simulink model "estimation_mdl"  (R2022b)
settings: Solver=FixedStepDiscrete  StartTime=0.0  StopTime=100  FixedStep=.1  RelTol=1e-3
values from neighbouring files (symbols this model uses):
  H = [1 3;4 0]    [estimation2d.m]    (also in estimation3d.m = [1 0 0;0 1 0;2 0 3]; filtering2_s.m = [1 3 -2;4 4 0]; tst1.m = [1 1])
  m = size(H,1)    [estimation2d.m]    (also in estimation3d.m; tst1.m)
  P0 = 1e2*eye(2)    [estimation2d.m]    (also in estimation3d.m = 1e2*eye(3); filtering1_s.m = V*diag([1 2])/V; filtering2_s.m = 1e1*eye(3); tst1.m = V*sqrt(D)*V.')
  Q = V*sqrt(D)    [estimation2d.m]    (also in estimation3d.m; ex_3_11.m = V*D12; filtering1_s.m; filtering2_s.m)
  R = (V /(sqrt(L))).'    [cellipse.m]    (also in estimation2d.m = V*D/V; estimation3d.m = V*D/V; filtering1_s.m = 3; filtering2_s.m = V*D/V)
  Ri = V*sqrt(L)    [cellipse.m]    (also in estimation2d.m = inv(R); estimation3d.m = inv(R); filtering1_s.m = inv(R); filtering2_s.m = inv(R))
  theta = 0:.05:2*pi    [cellipse.m]    (also in estimation2d.m = [8;-3]; estimation3d.m = [8;-3;4]; filtering1_s.m = [1.2, 3.4]; filtering2_s.m = [8;-3;15])
  xhat0 = [-5;-5]    [estimation2d.m]    (also in estimation3d.m = [-5;-5;0]; filtering1_s.m = [1;1]; filtering2_s.m = [0;0;0]; tst1.m)
undefined symbols (not defined in the file or in its folder): Discrete, Time
libraries: dspinverses x2, ctrlSharedLib x2
settings Model: Creator=hp_desktop  LastModifiedBy=hp_desktop

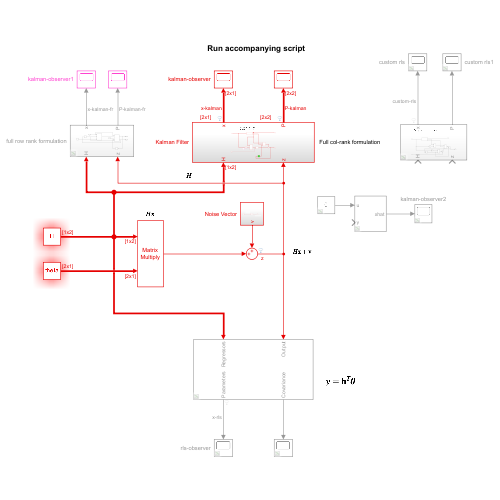
[thumbnail: Simulink's stored preview of the top-level diagram]
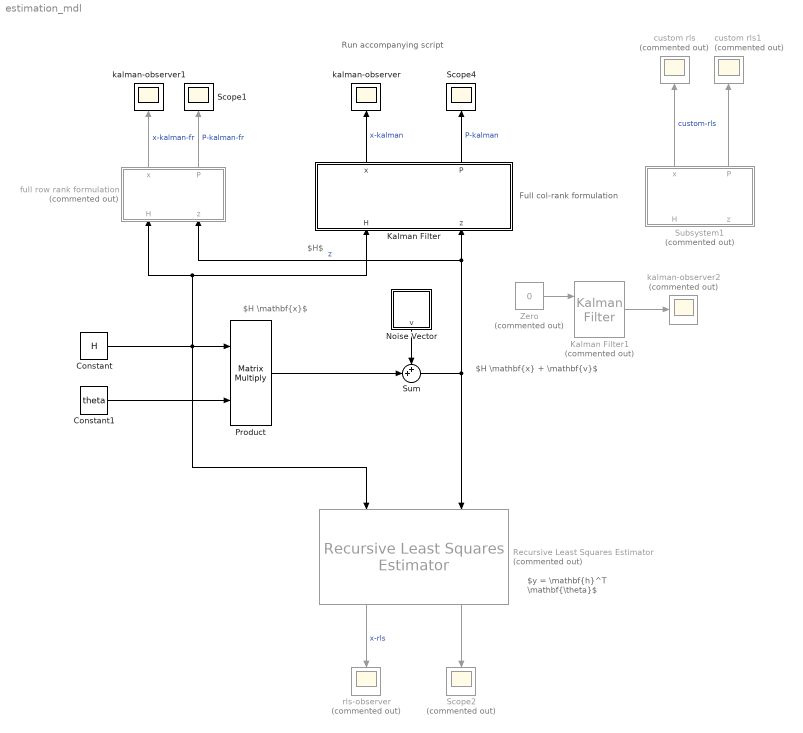
== system estimation_mdl ==
  note: Full col-rank formulation
  note: $H \mathbf{x}$
  note: Run accompanying script
  note: $y = \mathbf{h}^T \mathbf{\theta}$
  note: $H$
  note: $H \mathbf{x} + \mathbf{v}$
  Constant : Constant  Value=H  VectorParams1D=off  SampleTime=-1
  Constant1 : Constant  Value=theta  VectorParams1D=off  SampleTime=-1
  Kalman Filter : Subsystem
  Kalman Filter1 : ctrlSharedLib/Kalman Filter  Commented=on  TimeDomain=Discrete-Time  UseCurrentEstimator=on  ModelSource=Individual A, B, C, D matrices  ModelSourceVariable=ss(0.95,1,1,0,1)  A=[0 0;0 0]  B=[0;0]  C=H  D=zeros(m,1)  NumberOfStates=1  NumberOfInputs=1  NumberOfOutputs=1  InitialEstimateSource=Dialog  X0=xhat0  P0=10  UseK=off  UseGH=off  NumberOfProcessNoiseInputs=1  G=1  TimeInvariantG=on  H=0  TimeInvariantH=on  Q=0  TimeInvariantQ=on  R=R  TimeInvariantR=on  N=0  TimeInvariantN=on  AddInputPort=on  AddEnablePort=off  OutputEstimatedY=off  OutputP=off  Ts=-1
  Noise Vector : Subsystem
  Product : Product  Multiplication=Matrix(*)
  Recursive Least Squares Estimator : ctrlSharedLib/Recursive Least Squares Estimator  Commented=on  InitialEstimateSource=Internal  InitialParameterData=xhat0  P0=P0  InitialRegressors=0  InitialOutputs=0  History=Infinite  WindowLength=200  EstimationMethod=Kalman Filter  AdaptationParameter=0  HasTimeVaryingAdaptationParameter=off  NormalizationBias=eps  OutputError=off  OutputP=on  AddEnablePort=off  InputProcessing=Frame-based  Ts=-1
      settings: LibrarySourceBlock=slident/Estimators/Recursive Least Squares Estimator
  Scope1 : Scope
  Scope2 : Scope  Commented=on
  Scope4 : Scope
  Subsystem1 : Subsystem  Commented=on
      settings: PortSchema="{\"entries\":[{\"content\":{\"sides\":[{\"content\":{\"connectorIds\":[]},\"type\":\"ConnectorPlacement.EquallySpacedRectSide\",\"uuid\":\"bee4a480-fac8-4835-b5c1-70eb87c43e95\"},{\"content\":{\"connectorIds\":[],\"side\":\"RIGHT\"},\"type\":\"ConnectorPlacement.EquallySpacedRectSide\",\"uuid\":\"cb84ae2e-f606-4d86-aba4-d3e87a068395\"},{\"content\":{\"connectorIds\":[\"Out1\",\"Out2\"],\"side\":\"TOP\"},\"type\":\"ConnectorPlacement.EquallySpacedRectSide\",\"uuid\":\"f12c143d-ef46-4cd1-bb91-64452094197f\"},{\"content\":{\"connectorIds\":[\"In1\",\"In2\"],\"side\":\"BOTTOM\"},\"type\":\"ConnectorPlacement.EquallySpacedRectSide\",\"uuid\":\"568da4d9-a657-45a3-b36e-930d4945feb0\"}]},\"type\":\"ConnectorPlacement.EquallySpacedConnector\",\"uuid\":\"8fe02375-4d00-45c9-82ce-5394bc2c2119\"}],\"packageUris\":[\"http://schema.mathworks.com/mf0/Connector/R2020b\"],\"version\":\"1.0\"}"
  Sum : Sum  Inputs=++|
  Zero : Constant  Commented=on  Value=0  OutDataTypeStr=Inherit: Inherit via back propagation
  custom rls : Scope  Commented=on
  custom rls1 : Scope  Commented=on
  full row rank formulation : Subsystem  Commented=on
  kalman-observer : Scope
  kalman-observer1 : Scope
  kalman-observer2 : Scope  Commented=on
  rls-observer : Scope  Commented=on
  wires:
  Recursive Least Squares Estimator/1 -> rls-observer/1  "x-rls"
  Recursive Least Squares Estimator/2 -> Scope2/1
  Kalman Filter/1(x) -> kalman-observer/1  "x-kalman"
  Kalman Filter/2(P) -> Scope4/1  "P-kalman"
  Subsystem1/1(x) -> custom rls/1  "custom-rls"
  Subsystem1/2(P) -> custom rls1/1
  Sum/1 -> Recursive Least Squares Estimator/2, full row rank formulation/2(z), Kalman Filter/2(z)  "z"
  Constant/1 -> full row rank formulation/1(H), Kalman Filter/1(H), Product/1, Recursive Least Squares Estimator/1
  Constant1/1 -> Product/2
  Product/1 -> Sum/2
  Noise Vector/1(v) -> Sum/1
  full row rank formulation/1(x) -> kalman-observer1/1  "x-kalman-fr"
  full row rank formulation/2(P) -> Scope1/1  "P-kalman-fr"
  Zero/1 -> Kalman Filter1/1
  Kalman Filter1/1 -> kalman-observer2/1

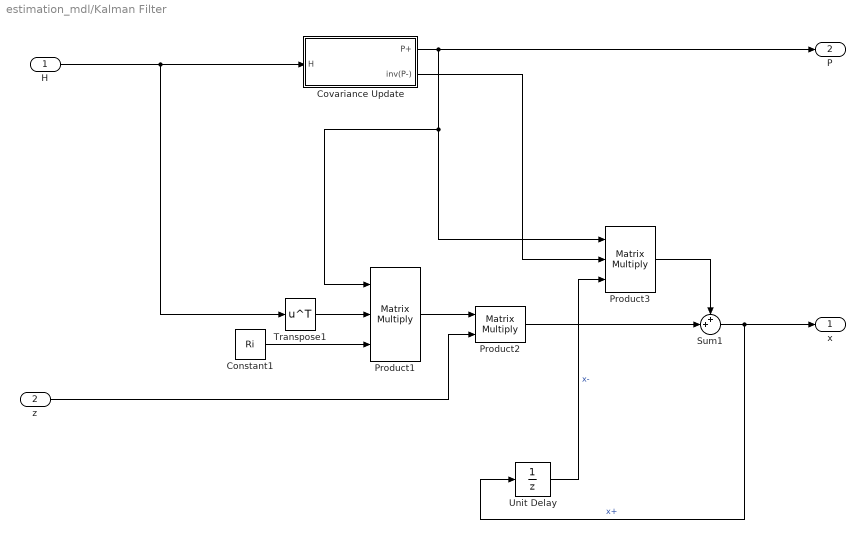
== system estimation_mdl/Kalman Filter ==
  H : Inport
  z : Inport  Port=2
  Constant1 : Constant  Value=Ri  VectorParams1D=off
  Covariance Update : Subsystem
  Product1 : Product  Inputs=3  Multiplication=Matrix(*)
  Product2 : Product  Multiplication=Matrix(*)
  Product3 : Product  Inputs=3  Multiplication=Matrix(*)
  Sum1 : Sum  Inputs=++|
  Transpose1 : Math  Operator=transpose
  Unit Delay : UnitDelay  InitialCondition=xhat0  SampleTime=-1  HasFrameUpgradeWarning=on
  x : Outport
  P : Outport  Port=2
  wires:
  Sum1/1 -> Unit Delay/1, x/1  "x+"
  Transpose1/1 -> Product1/2
  Constant1/1 -> Product1/3
  Product1/1 -> Product2/1
  z/1 -> Product2/2
  Unit Delay/1 -> Product3/3  "x-"
  Product3/1 -> Sum1/1
  Product2/1 -> Sum1/2
  H/1 -> Transpose1/1, Covariance Update/1(H)
  Covariance Update/1(P+) -> P/1, Product1/1, Product3/1
  Covariance Update/2(inv(P-)) -> Product3/2

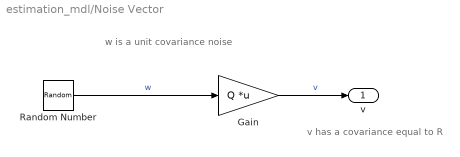
== system estimation_mdl/Noise Vector ==
  note: w is a
      | unit covariance noise
  note: v has a covariance equal to R
  Gain : Gain  Gain=Q  Multiplication=Matrix(K*u)
  Random Number : RandomNumber  Seed=randi(1e8, m,1)  SampleTime=.1  VectorParams1D=off
  v : Outport
  wires:
  Random Number/1 -> Gain/1  "w"
  Gain/1 -> v/1  "v"

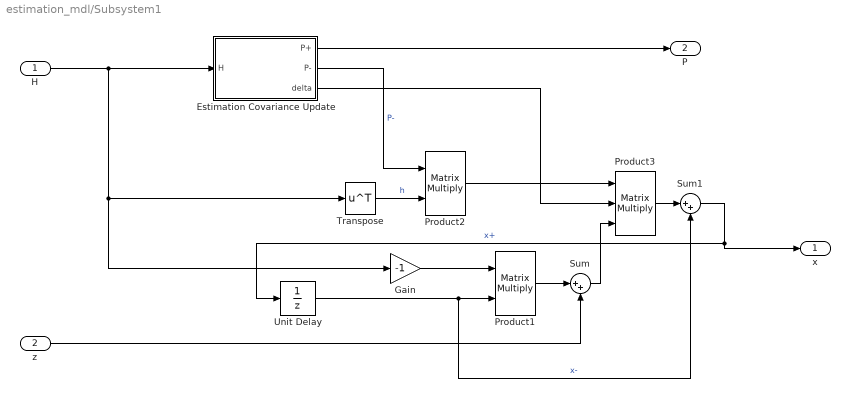
== system estimation_mdl/Subsystem1 ==
  H : Inport
  z : Inport  Port=2
  Estimation Covariance Update : Subsystem
  Gain : Gain  Gain=-1
  Product1 : Product  Multiplication=Matrix(*)
  Product2 : Product  Multiplication=Matrix(*)
  Product3 : Product  Inputs=3  Multiplication=Matrix(*)
  Sum : Sum  Inputs=|++
  Sum1 : Sum  Inputs=|++
  Transpose : Math  Operator=transpose
  Unit Delay : UnitDelay  SampleTime=-1  HasFrameUpgradeWarning=on
  x : Outport
  P : Outport  Port=2
  wires:
  Estimation Covariance Update/1(P+) -> P/1
  Unit Delay/1 -> Sum1/2, Product1/2  "x-"
  Sum1/1 -> x/1, Unit Delay/1  "x+"
  Transpose/1 -> Product2/2  "h"
  Product2/1 -> Product3/1
  Estimation Covariance Update/2(P-) -> Product2/1  "P-"
  H/1 -> Estimation Covariance Update/1(H), Gain/1, Transpose/1
  Gain/1 -> Product1/1
  Product1/1 -> Sum/1
  z/1 -> Sum/2
  Estimation Covariance Update/3(delta) -> Product3/2
  Sum/1 -> Product3/3
  Product3/1 -> Sum1/1

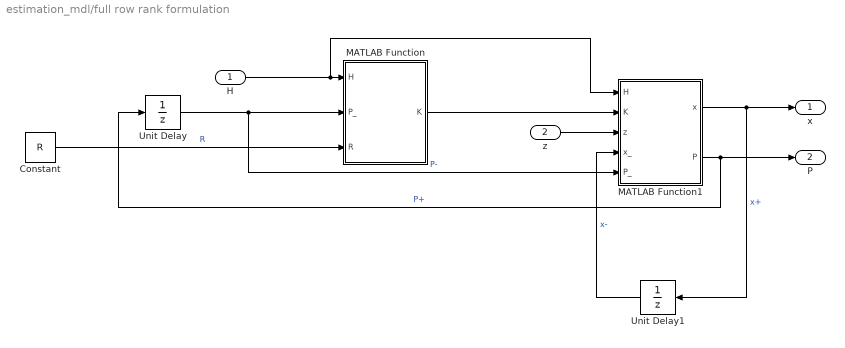
== system estimation_mdl/full row rank formulation ==
  H : Inport
  z : Inport  Port=2
  Constant : Constant  Value=R  VectorParams1D=off
  MATLAB Function : MATLAB Function  TreatAsAtomicUnit=on
  MATLAB Function1 : MATLAB Function  TreatAsAtomicUnit=on
  Unit Delay : UnitDelay  InitialCondition=P0  SampleTime=-1  HasFrameUpgradeWarning=on
  Unit Delay1 : UnitDelay  InitialCondition=xhat0  SampleTime=-1  HasFrameUpgradeWarning=on
  x : Outport
  P : Outport  Port=2
  wires:
  H/1 -> MATLAB Function1/1(H), MATLAB Function/1(H)
  MATLAB Function1/2(P) -> Unit Delay/1, P/1  "P+"
  Unit Delay/1 -> MATLAB Function/2(P_), MATLAB Function1/5(P_)  "P-"
  Constant/1 -> MATLAB Function/3(R)  "R"
  Unit Delay1/1 -> MATLAB Function1/4(x_)  "x-"
  MATLAB Function1/1(x) -> x/1, Unit Delay1/1  "x+"
  z/1 -> MATLAB Function1/3(z)
  MATLAB Function/1(K) -> MATLAB Function1/2(K)

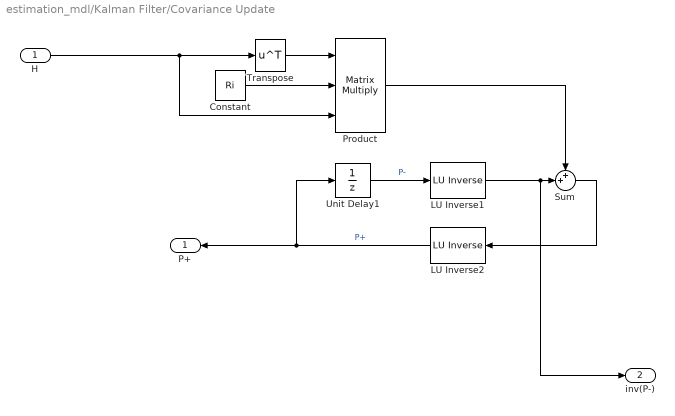
== system estimation_mdl/Kalman Filter/Covariance Update ==
  H : Inport
  " LU Inverse1" : dspinverses/ LU Inverse
  " LU Inverse2" : dspinverses/ LU Inverse
  Constant : Constant  Value=Ri  VectorParams1D=off
  Product : Product  Inputs=3  Multiplication=Matrix(*)
  Sum : Sum  Inputs=++|
  Transpose : Math  Operator=transpose
  Unit Delay1 : UnitDelay  InitialCondition=P0  SampleTime=-1  HasFrameUpgradeWarning=on
  P+ : Outport
  inv(P-) : Outport  Port=2
  wires:
  H/1 -> Product/3, Transpose/1
  Transpose/1 -> Product/1
  " LU Inverse1"/1 -> inv(P-)/1, Sum/2
  " LU Inverse2"/1 -> Unit Delay1/1, P+/1  "P+"
  Constant/1 -> Product/2
  Product/1 -> Sum/1
  Unit Delay1/1 -> " LU Inverse1"/1  "P-"
  Sum/1 -> " LU Inverse2"/1

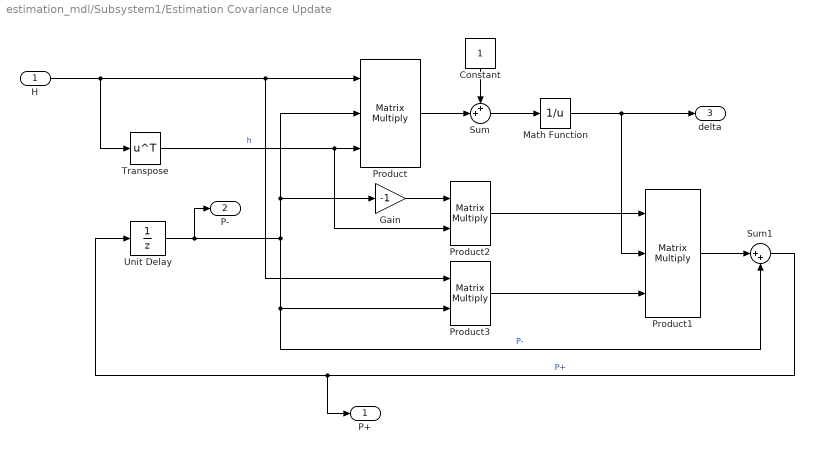
== system estimation_mdl/Subsystem1/Estimation Covariance Update ==
  H : Inport
  Constant : Constant
  Gain : Gain  Gain=-1
  Math Function : Math  Operator=reciprocal
  Product : Product  Inputs=3  Multiplication=Matrix(*)
  Product1 : Product  Inputs=3  Multiplication=Matrix(*)
  Product2 : Product  Multiplication=Matrix(*)
  Product3 : Product  Multiplication=Matrix(*)
  Sum : Sum  Inputs=++|
  Sum1 : Sum  Inputs=|++
  Transpose : Math  Operator=transpose
  Unit Delay : UnitDelay  InitialCondition=diag([1 2])  SampleTime=-1  HasFrameUpgradeWarning=on
  P+ : Outport
  P- : Outport  Port=2
  delta : Outport  Port=3
  wires:
  Sum1/1 -> P+/1, Unit Delay/1  "P+"
  Unit Delay/1 -> P-/1, Sum1/2, Product3/2, Product/2, Gain/1  "P-"
  H/1 -> Transpose/1, Product3/1, Product/1
  Transpose/1 -> Product/3, Product2/2  "h"
  Product/1 -> Sum/2
  Constant/1 -> Sum/1
  Sum/1 -> Math Function/1
  Gain/1 -> Product2/1
  Product2/1 -> Product1/1
  Math Function/1 -> delta/1, Product1/2
  Product3/1 -> Product1/3
  Product1/1 -> Sum1/1

== matlab function estimation_mdl/full row rank formulation/MATLAB Function1 ==
  data: H input; K input; z input; x_ input; P_ input; x output; P output
function [x,P] = fcn(H, K, z, x_, P_)

x = x_ + K*(z-H*x_);
P = P_ -K*H*P_;

end

== matlab function estimation_mdl/full row rank formulation/MATLAB Function ==
  data: H input; P_ input; K output; R input
function K = fcn(H, P_, R)

K = P_ * H.' /(H*P_*H.' + R);

end
